simulink model "closedloopmodel_saturation_control101"  (R2025b)
settings: Solver=VariableStepAuto  StartTime=0.0  StopTime=stoptime  RelTol=1e-3
undefined symbols (not defined in the file or in its folder): den, gain, Kfeedback, num, target, umax, umin
settings Model: Creator=Anthony Rossiter  LastModifiedBy=Anthony Rossiter

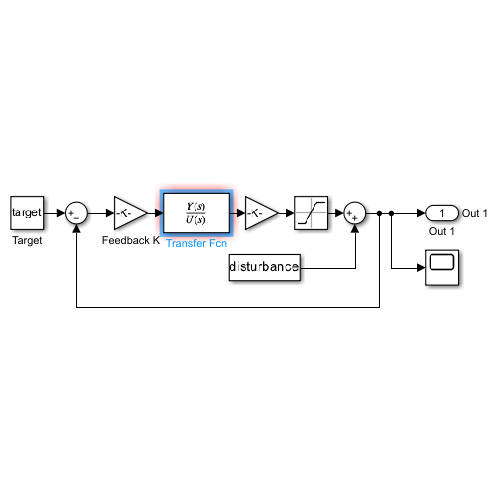
[thumbnail: Simulink's stored preview of the top-level diagram]
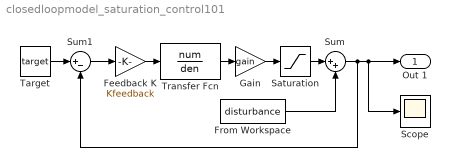
== system closedloopmodel_saturation_control101 ==
  Feedback K : Gain  Gain=Kfeedback
  From Workspace : FromWorkspace  VariableName=disturbance
  Gain : Gain  Gain=gain
  Saturation : Saturate  UpperLimit=umax  LowerLimit=umin
  Scope : Scope
  Sum : Sum  Inputs=|++
  Sum1 : Sum  Inputs=|+-
  Target : Constant  Value=target
  Transfer Fcn : TransferFcn  Numerator=num  Denominator=den
  Out 1 : Outport  SignalName=Out 1
  wires:
  Gain/1 -> Saturation/1
  Transfer Fcn/1 -> Gain/1
  Saturation/1 -> Sum/1
  Sum/1 -> Sum1/2, Scope/1, Out 1/1
  From Workspace/1 -> Sum/2
  Target/1 -> Sum1/1
  Sum1/1 -> Feedback K/1
  Feedback K/1 -> Transfer Fcn/1
